simulink model "penduloLQR"  (Simulink 7.3)
settings: Solver=ode45  StartTime=0.0  StopTime=10  RelTol=1e-3
values from neighbouring files (symbols this model uses):
  K = lqr(A,B,Q,R)    [LQR.m]    (also in bestQ.m = setK_lqr(Q_i); graficosPenduloReal.m = setK_lqr(Q_optimo))
libraries: simulink x6
settings Model: Creator=Daniel  LastModifiedBy=Daniel

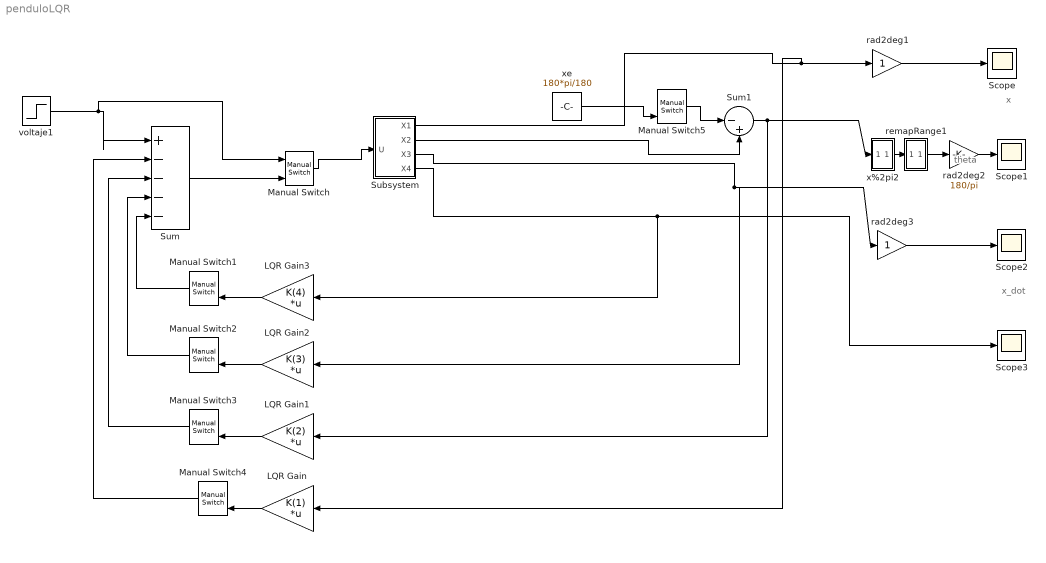
== system penduloLQR ==
  note: x
  note: theta
  note: x_dot
  LQR Gain : Gain  Gain=K(1)  Multiplication=Matrix(K*u)  SaturateOnIntegerOverflow=on  OutDataTypeStr=Inherit: Same as input  ParamDataTypeStr=Inherit: Same as input
  LQR Gain1 : Gain  Gain=K(2)  Multiplication=Matrix(K*u)  SaturateOnIntegerOverflow=on  OutDataTypeStr=Inherit: Same as input  ParamDataTypeStr=Inherit: Same as input
  LQR Gain2 : Gain  Gain=K(3)  Multiplication=Matrix(K*u)  SaturateOnIntegerOverflow=on  OutDataTypeStr=Inherit: Same as input  ParamDataTypeStr=Inherit: Same as input
  LQR Gain3 : Gain  Gain=K(4)  Multiplication=Matrix(K*u)  SaturateOnIntegerOverflow=on  OutDataTypeStr=Inherit: Same as input  ParamDataTypeStr=Inherit: Same as input
  Manual Switch : simulink/Signal Routing/Manual Switch  SystemSampleTime=-1  sw=1  action=0  varsize=off
  Manual Switch{1..5} (5 alike) : simulink/Signal Routing/Manual Switch  SystemSampleTime=-1  sw=0  action=0  varsize=off
  Scope{,1..3} (4 alike) : Scope
      Scope settings: YMin=-2e+007  YMax=-4e+006
      Scope1 settings: YMin=89.1  YMax=90.9
      Scope2 settings: YMin=2.0025e+016  YMax=2.0325e+016  SaveName=ScopeData2
      Scope3 settings: YMin=-1.1e+007  YMax=1.1e+007  SaveName=ScopeData3
  Subsystem : Subsystem
  Sum : Sum  Inputs=|+----
  Sum1 : Sum  Inputs=|-+
  rad2deg1 : Gain  SaturateOnIntegerOverflow=on  OutDataTypeStr=Inherit: Same as input  ParamDataTypeStr=Inherit: Same as input
  rad2deg2 : Gain  Gain=180/pi  SaturateOnIntegerOverflow=on  OutDataTypeStr=Inherit: Same as input  ParamDataTypeStr=Inherit: Same as input
  rad2deg3 : Gain  SaturateOnIntegerOverflow=on  OutDataTypeStr=Inherit: Same as input  ParamDataTypeStr=Inherit: Same as input
  remapRange1 : Stateflow chart  TreatAsAtomicUnit=on
  voltaje1 : Step  Time=0  After=2.5  SampleTime=0.1
  x%2pi2 : Stateflow chart  TreatAsAtomicUnit=on
  xe : Constant  Value=180*pi/180  OutDataType=fixdt(1, 16)  OutScaling=2^0
  wires:
  rad2deg3/1 -> Scope2/1
  Subsystem/3(X3) -> LQR Gain2/1, rad2deg3/1
  rad2deg1/1 -> Scope/1
  Subsystem/1(X1) -> rad2deg1/1, LQR Gain/1
  LQR Gain3/1 -> Manual Switch1/2
  LQR Gain2/1 -> Manual Switch2/2
  LQR Gain1/1 -> Manual Switch3/2
  Manual Switch/1 -> Subsystem/1(U)
  Subsystem/4(X4) -> LQR Gain3/1, Scope3/1
  LQR Gain/1 -> Manual Switch4/2
  x%2pi2/1(y) -> remapRange1/1(value)
  remapRange1/1(y) -> rad2deg2/1
  Manual Switch1/1 -> Sum/5
  Manual Switch3/1 -> Sum/3
  Manual Switch4/1 -> Sum/2
  voltaje1/1 -> Sum/1, Manual Switch/1
  Sum/1 -> Manual Switch/2
  Manual Switch2/1 -> Sum/4
  rad2deg2/1 -> Scope1/1
  Subsystem/2(X2) -> Sum1/2
  Sum1/1 -> x%2pi2/1(u), LQR Gain1/1
  Manual Switch5/1 -> Sum1/1
  xe/1 -> Manual Switch5/2

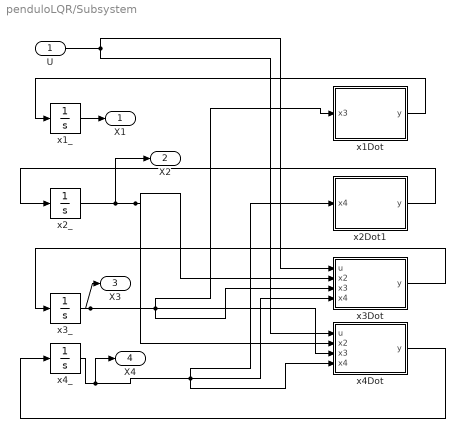
== system penduloLQR/Subsystem ==
  U : Inport
  x1Dot : Stateflow chart
  x1_ : Integrator  UpperSaturationLimit=2  LowerSaturationLimit=-2
  x2Dot1 : Stateflow chart
  x2_ : Integrator  InitialCondition=170*pi/180  UpperSaturationLimit=100  LowerSaturationLimit=-100
  x3Dot : Stateflow chart
  x3_ : Integrator  UpperSaturationLimit=10  LowerSaturationLimit=-10
  x4Dot : Stateflow chart
  x4_ : Integrator  UpperSaturationLimit=60  LowerSaturationLimit=-60
  X1 : Outport
  X2 : Outport  Port=2
  X3 : Outport  Port=3
  X4 : Outport  Port=4
  wires:
  x1Dot/1(y) -> x1_/1
  x2Dot1/1(y) -> x2_/1
  x3Dot/1(y) -> x3_/1
  x3_/1 -> X3/1, x1Dot/1(x3), x4Dot/3(x3), x3Dot/3(x3)
  x4Dot/1(y) -> x4_/1
  x4_/1 -> X4/1, x2Dot1/1(x4), x3Dot/4(x4), x4Dot/4(x4)
  x1_/1 -> X1/1
  U/1 -> x4Dot/1(u), x3Dot/1(u)
  x2_/1 -> X2/1, x3Dot/2(x2), x4Dot/2(x2)

== matlab function Subsystem/x3Dot ==
  data: u input double; y output double; x2 input double; x3 input double; x4 input double
function y = x3Dot(u,x2,x3,x4)
I = 0.0138;
g = 9.81;
b = 0.05;
l = 0.3213;
m = 0.104;
M = 0.768;

y =  (I + m*(l^2))*  ( (1.88*u -4.7 + m*l*(x4^2)*sin(x2) -(b+0.548)*x3 + ((m^2)*(l^2)*g*sin(2*x2)/(2*(I+m*(l^2)))) ) /  ((M+m)*(I+m*(l^2)) - (m^2)*(l^2)*((cos(x2))^2))) ;
end

== matlab function Subsystem/x4Dot ==
  data: u input double; y output double; x2 input double; x3 input double; x4 input double
function y = x4Dot(u,x2,x3,x4)
I = 0.0138;
g = 9.81;
b = 0.05;
l = 0.3213;
m = 0.104;
M = 0.768;

y =m*l*(( (1.88*u -4.7 + m*l*(x4^2)*sin(x2) -(b+0.548)*x3)*cos(x2) + (M+m)*g*sin(x2)) /  ((m^2)*(l^2)*((cos(x2))^2)- (M+m)*(I+m*(l^2)))) ;
end

== matlab function remapRange1 ==
  data: value input double; y output double
function y = remapRange(value)
    scaleFactor = pi/180;
    if (value>180*scaleFactor)
        %constants
        fromLow = 181*scaleFactor;
        fromHigh = 360*scaleFactor;
        toLow = -179*scaleFactor;
        toHigh = 0*scaleFactor;
        %calculations
        new_range = toHigh-toLow;
        old_range = fromHigh - fromLow;
        new_value = (new_range/old_range)*(value-fromLow)+toLow;
        y = new_value;
    else
        y = value;
    end
        
end

== matlab function x%2pi2 ==
  data: u input double; y output double
function y = fcn(u)
%#codegen
    y = mod(u,2*pi);
end

== matlab function Subsystem/x1Dot ==
  data: y output double; x3 input double
function y = x1Dot(x3)
y = x3;
end

== matlab function Subsystem/x2Dot1 ==
  data: y output double; x4 input double
function y = x2Dot(x4)
y = x4;
end
